simulink library "Tire_2x"  (R2026a)
settings: Solver=VariableStepAuto
undefined symbols (not defined in the file): rhs_tire, tir_index, Tire, X, Y, Z
libraries: Tire_1x x2, sm_lib x2
Description:
  | Copyright 2020-2024 The MathWorks, Inc.
settings Model: Creator=smiller  LastModifiedBy=andrei

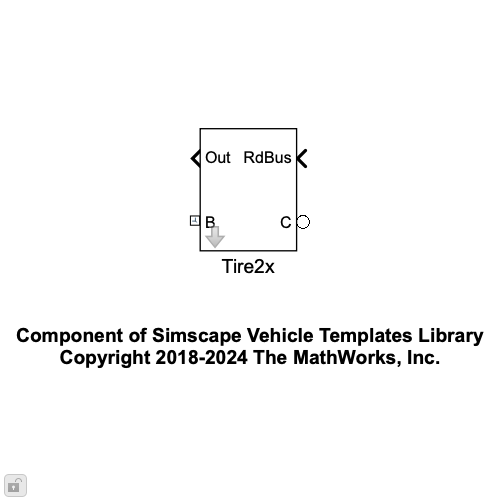
[thumbnail: Simulink's stored preview of the top-level diagram]
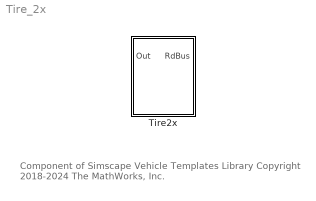
== system Tire_2x ==
  note: Component of Simscape Vehicle Templates Library
      | Copyright 2018-2024 The MathWorks, Inc.
  Tire2x : Subsystem  VariantControl=Tire2x  mask{popup_leftRight=Right, tir_index=tir_index, TireInner=Tire.TireInner, TireOuter=Tire.TireOuter}
      mask prompts: popup_leftRight "Left/Right"; tir_index "Tire Index"; TireInner "Tire Inner (structure)"; TireOuter "Tire Outer (structure)"
      mask init:
      | curblk = gcb;
      | 
      | if(popup_leftRight == 1)
      |     set_param([curblk '/Tire Inner'],'popup_leftRight','Left');
      |     set_param([curblk '/Tire Outer'],'popup_leftRight','Left');
      | elseif(popup_leftRight == 2)
      |     set_param([curblk '/Tire Inner'],'popup_leftRight','Right');
      |     set_param([curblk '/Tire Outer'],'popup_leftRight','Right');
      | end
      mask TypeOptions popup_leftRight: Left | Right
      mask DialogControl cont_tire_mfeval Prompt: Tire

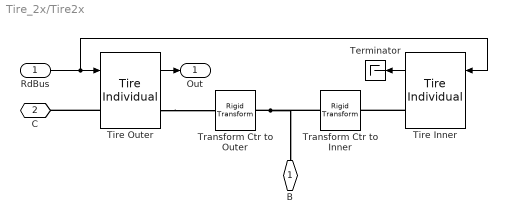
== system Tire_2x/Tire2x ==
  RdBus : Inport
  Terminator : Terminator
  Tire Inner : Tire_1x/Tire Individual  Tag=PublishSubsystem  VariantControl=Variant1  LabelModeActiveChoice=MFMbody  popup_leftRight=Right  tir_index=tir_index+1  Tire=TireInner  VariantLabel=TireInner.class.Value
      settings: AttributesFormatString=%<ActiveVariant>
  Tire Outer : Tire_1x/Tire Individual  Tag=PublishSubsystem  VariantControl=Variant1  LabelModeActiveChoice=MFMbody  popup_leftRight=Right  tir_index=tir_index  Tire=TireOuter  VariantLabel=TireOuter.class.Value
      settings: AttributesFormatString=%<ActiveVariant>
  Transform Ctr to Inner : sm_lib/Frames and Transforms/Rigid Transform  RotationMethod=None  FollAlignAxisA=+X  BaseAlignAxisA=+Y  FollAlignAxisB=+Y  BaseAlignAxisB=+Z  RotationStandardAxis=+Z  RotationAngle=0.0  RotationAngleUnits=deg  RotationArbitraryAxis=[0 0 1]  RotationSequenceAxes=FollowerAxes  RotationSequence=XYX  RotationSequenceAngles=[0 0 0]  RotationSequenceAnglesUnits=deg  RotationMatrix=[1 0 0; 0 1 0; 0 0 1]  Quaternion=[1 0 0 0]  TranslationMethod=StandardAxis  TranslationCartesianOffset=[0 0 0]  TranslationCartesianOffsetUnits=m  TranslationStandardAxis=-Z  TranslationStandardOffset=Tire.xOffset.Value/2*rhs_tire  TranslationStandardOffsetUnits=m  TranslationROffset=0  TranslationROffsetUnits=m  TranslationThetaOffset=0  TranslationThetaOffsetUnits=deg  TranslationZOffset=0  TranslationZOffsetUnits=m
  Transform Ctr to Outer : sm_lib/Frames and Transforms/Rigid Transform  RotationMethod=None  FollAlignAxisA=+X  BaseAlignAxisA=+Y  FollAlignAxisB=+Y  BaseAlignAxisB=+Z  RotationStandardAxis=+Z  RotationAngle=0.0  RotationAngleUnits=deg  RotationArbitraryAxis=[0 0 1]  RotationSequenceAxes=FollowerAxes  RotationSequence=XYX  RotationSequenceAngles=[0 0 0]  RotationSequenceAnglesUnits=deg  RotationMatrix=[1 0 0; 0 1 0; 0 0 1]  Quaternion=[1 0 0 0]  TranslationMethod=StandardAxis  TranslationCartesianOffset=[0 0 0]  TranslationCartesianOffsetUnits=m  TranslationStandardAxis=+Z  TranslationStandardOffset=Tire.xOffset.Value/2*rhs_tire  TranslationStandardOffsetUnits=m  TranslationROffset=0  TranslationROffsetUnits=m  TranslationThetaOffset=0  TranslationThetaOffsetUnits=deg  TranslationZOffset=0  TranslationZOffsetUnits=m
  B : PMIOPort  Side=Right
  C : PMIOPort  Port=2  Side=Left
  Out : Outport  VectorParamsAs1DForOutWhenUnconnected=off
  wires:
  Tire Inner/1 -> Terminator/1
  Tire Outer/1 -> Out/1
  RdBus/1 -> Tire Inner/1, Tire Outer/1
  connections:
  Tire Outer/RConn1 -- Transform Ctr to Outer/RConn1
  Tire Inner/RConn1 -- Transform Ctr to Inner/RConn1
  Tire Outer/LConn1 -- C/RConn1
  Transform Ctr to Outer/LConn1 -- B/RConn1 -- Transform Ctr to Inner/LConn1
